simulink model "Additional"  (R2013b)
settings: Solver=ode45  StartTime=0.0  StopTime=200  RelTol=1e-3
settings Model: Creator=sz609516  LastModifiedBy=tth-sza
settings DebuggingCC: StateNameClashWarn=warning

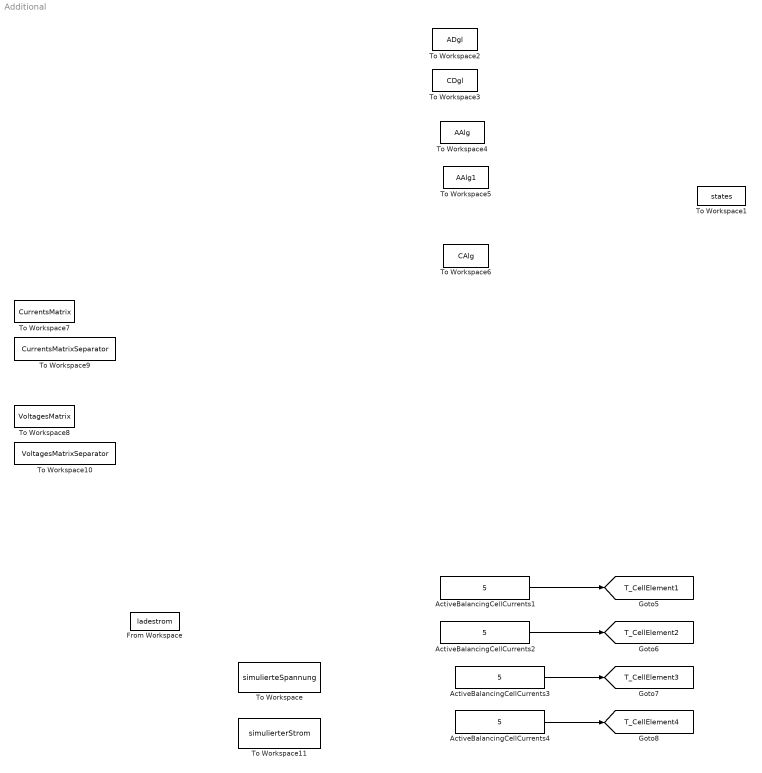
== system Additional ==
  ActiveBalancingCellCurrents{1..4} (4 alike) : Constant  Value=5
  From Workspace : FromWorkspace  VariableName=ladestrom  SampleTime=0
  To Workspace : ToWorkspace  VariableName=simulierteSpannung  SampleTime=-1  SaveFormat=Structure With Time
  To Workspace1 : ToWorkspace  VariableName=states  SampleTime=1.0  SaveFormat=Structure With Time
  To Workspace10 : ToWorkspace  VariableName=VoltagesMatrixSeparator  SampleTime=1.0  SaveFormat=Structure With Time
      settings: MaxDataPoints=1
  To Workspace11 : ToWorkspace  VariableName=simulierterStrom  SampleTime=-1  SaveFormat=Structure With Time
  To Workspace2 : ToWorkspace  VariableName=ADgl  SampleTime=1.0  SaveFormat=Structure With Time
  To Workspace3 : ToWorkspace  VariableName=CDgl  SampleTime=1.0  SaveFormat=Structure With Time
  To Workspace4 : ToWorkspace  VariableName=AAlg  SampleTime=1.0  SaveFormat=Structure With Time
  To Workspace5 : ToWorkspace  VariableName=AAlg1  SampleTime=1.0  SaveFormat=Structure With Time
  To Workspace6 : ToWorkspace  VariableName=CAlg  SampleTime=1.0  SaveFormat=Structure With Time
  To Workspace7 : ToWorkspace  VariableName=CurrentsMatrix  SampleTime=1.0  SaveFormat=Structure With Time
  To Workspace8 : ToWorkspace  VariableName=VoltagesMatrix  SampleTime=1.0  SaveFormat=Structure With Time
  To Workspace9 : ToWorkspace  VariableName=CurrentsMatrixSeparator  SampleTime=1.0  SaveFormat=Structure With Time
      settings: MaxDataPoints=1
  tag scope: T_CellElement1=global, T_CellElement2=global, T_CellElement3=global, T_CellElement4=global
  wires:
  ActiveBalancingCellCurrents4/1 -> [T_CellElement4]
  ActiveBalancingCellCurrents3/1 -> [T_CellElement3]
  ActiveBalancingCellCurrents2/1 -> [T_CellElement2]
  ActiveBalancingCellCurrents1/1 -> [T_CellElement1]
